simulink model "State_Feedback_NON_Linear_ROS"  (R2022b)
settings: Solver=FixedStepAuto  StartTime=0.0  StopTime=45  FixedStep=0.02  RelTol=1e-3
undefined symbols (not defined in the file): unicycle, X, Y
libraries: robotlib x3, simulink_extras x2
settings Model: Creator=Musta  LastModifiedBy=Musta
settings OptimizationCC: EnhancedBackFolding=on  PassReuseOutputArgsAs=Individual arguments  ZeroExternalMemoryAtStartup=off  ZeroInternalMemoryAtStartup=off  MaxStackSize=64  OptimizeBlockOrder=speed  DifferentSizesBufferReuse=on  OptimizationCustomize=off  EfficientTunableParamExpr=on
settings DebuggingCC: ParameterTunabilityLossMsg=error
settings HardwareCC: ProdBitPerPointer=32  ProdBitPerSizeT=32  ProdBitPerPtrDiffT=32  ProdLargestAtomicFloat=None  ProdIntDivRoundTo=Undefined  ProdEndianess=Unspecified  ProdWordSize=32  ProdHWDeviceType=Generic->Unspecified (assume 32-bit Generic)
settings SFSimCC: MATLABDynamicMemAlloc=off
settings RTWCC: Description=Embedded Coder  SystemTargetFile=ert.tlc  HardwareBoard=Robot Operating System (ROS)  TLCOptions="-aInlineSetEventsForThisBaseRateFcn=TLC_FALSE -aSuppressMultiTaskScheduler=TLC_FALSE  -aRateBasedStepFcn=0"  TemplateMakefile=ert_default_tmf  Toolchain=Catkin  TargetLang=C++
settings CodeAppCC: ForceParamTrailComments=on  IgnoreCustomStorageClasses=off  OperatorAnnotations=on  SimulinkDataObjDesc=on  SFDataObjDesc=on  InsertBlockDesc=on

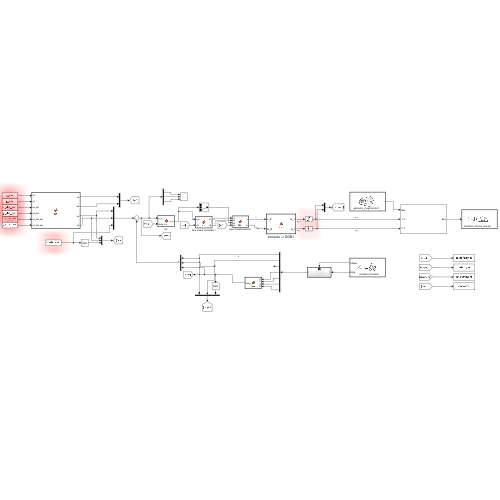
[thumbnail: Simulink's stored preview of the top-level diagram]
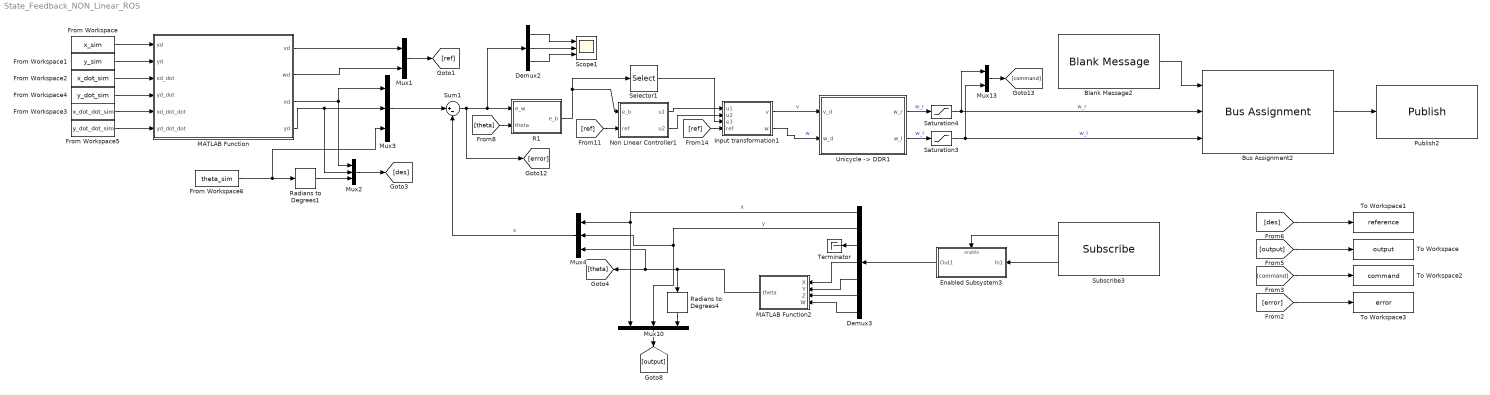
== system State_Feedback_NON_Linear_ROS ==
  Blank Message2 : robotlib/Blank Message  messageClass=Message  entityType=geometry_msgs/Vector3  messageType=geometry_msgs/Vector3  SampleTime=0.02  legacyBusStruct=off
      settings: LibrarySourceBlock=roslib/ROS/Blank Message
  Bus Assignment2 : BusAssignment  AssignedSignals=X,Y
  Demux2 : Demux  Outputs=3
  Demux3 : Demux  Outputs=7
  Enabled Subsystem3 : Subsystem  TreatAsAtomicUnit=on
  From Workspace : FromWorkspace  VariableName=x_sim
  From Workspace1 : FromWorkspace  VariableName=y_sim
  From Workspace2 : FromWorkspace  VariableName=x_dot_sim
  From Workspace3 : FromWorkspace  VariableName=x_dot_dot_sim
  From Workspace4 : FromWorkspace  VariableName=y_dot_sim
  From Workspace5 : FromWorkspace  VariableName=y_dot_dot_sim
  From Workspace6 : FromWorkspace  VariableName=theta_sim
  Input transformation1 : MATLAB Function  TreatAsAtomicUnit=on
  MATLAB Function : MATLAB Function  TreatAsAtomicUnit=on
  MATLAB Function2 : MATLAB Function  TreatAsAtomicUnit=on
  Mux1 : Mux  Inputs=2
  Mux{2..4,10} (4 alike) : Mux  Inputs=3
  Mux13 : Mux  Inputs=2
  Non Linear Controller1 : MATLAB Function  TreatAsAtomicUnit=on
  Publish2 : robotlib/Publish  topicSource=Select from ROS network  topic=/turtlebot_03/cmd_wheels  messageType=geometry_msgs/Vector3  legacyBusStruct=off  messageQueueLength=1
      settings: LibrarySourceBlock=roslib/ROS/Publish
  R1 : MATLAB Function  TreatAsAtomicUnit=on
  Radians to Degrees1 : simulink_extras/Transformations/Radians to Degrees
  Radians to Degrees4 : simulink_extras/Transformations/Radians to Degrees
  Saturation3 : Saturate  UpperLimit=unicycle.omegaWheelMax  LowerLimit=unicycle.omegaWheelMin
  Saturation4 : Saturate  UpperLimit=unicycle.omegaWheelMax  LowerLimit=unicycle.omegaWheelMin
  Scope1 : Scope  NumInputPorts=3
  Selector1 : Selector  InputPortWidth=3  IndexOptions=Index vector (dialog)  Indices=3  OutputSizes=1
  Subscribe3 : robotlib/Subscribe  topicSource=Select from ROS network  topic=/turtlebot_03/odom  messageType=nav_msgs/Odometry  SampleTime=0.02  legacyBusStruct=off  messageQueueLength=1
      settings: LibrarySourceBlock=roslib/ROS/Subscribe
  Sum1 : Sum  Inputs=|+-
  Terminator : Terminator
  To Workspace : ToWorkspace  VariableName=output  SaveFormat=Structure With Time  SampleTime=-1
  To Workspace1 : ToWorkspace  VariableName=reference  SaveFormat=Structure With Time  SampleTime=-1
  To Workspace2 : ToWorkspace  VariableName=command  SaveFormat=Structure With Time  SampleTime=-1
  To Workspace3 : ToWorkspace  VariableName=error  SaveFormat=Structure With Time  SampleTime=-1
  "Unicycle -> DDR1" : MATLAB Function  TreatAsAtomicUnit=on
  wires:
  [command] -> To Workspace2/1
  [des] -> To Workspace1/1
  [output] -> To Workspace/1
  [error] -> To Workspace3/1
  Subscribe3/2 -> Enabled Subsystem3/1(In1)
  Subscribe3/1 -> Enabled Subsystem3/Enable
  Demux2/2 -> Scope1/2
  Non Linear Controller1/1(u1) -> Input transformation1/1(u1)
  [theta] -> R1/2(theta)
  Demux2/1 -> Scope1/1
  Sum1/1 -> [error], R1/1(e_w), Demux2/1
  Blank Message2/1 -> Bus Assignment2/1
  Input transformation1/1(v) -> "Unicycle -> DDR1"/1(v_d)  "v"
  Selector1/1 -> Input transformation1/3(e3)
  [ref] -> Non Linear Controller1/2(ref)
  Input transformation1/2(w) -> "Unicycle -> DDR1"/2(w_d)  "w"
  Mux13/1 -> [command]
  Saturation4/1 -> Bus Assignment2/2, Mux13/1  "w_r"
  Demux2/3 -> Scope1/3
  Saturation3/1 -> Bus Assignment2/3, Mux13/2  "w_l"
  R1/1(e_b) -> Non Linear Controller1/1(e_b), Selector1/1
  "Unicycle -> DDR1"/2(w_l) -> Saturation3/1  "w_l"
  [ref] -> Input transformation1/4(ref)
  Bus Assignment2/1 -> Publish2/1
  "Unicycle -> DDR1"/1(w_r) -> Saturation4/1  "w_r"
  Non Linear Controller1/2(u2) -> Input transformation1/2(u2)
  From Workspace/1 -> MATLAB Function/1("xd ")
  From Workspace6/1 -> Radians to Degrees1/1, Mux3/3
  Mux2/1 -> [des]
  Mux1/1 -> [ref]
  MATLAB Function/2(wd) -> Mux1/2
  From Workspace1/1 -> MATLAB Function/2("yd ")
  From Workspace3/1 -> MATLAB Function/5(xd_dot_dot)
  From Workspace5/1 -> MATLAB Function/6(yd_dot_dot)
  MATLAB Function/4(yd) -> Mux2/2, Mux3/2
  From Workspace2/1 -> MATLAB Function/3(xd_dot)
  From Workspace4/1 -> MATLAB Function/4(yd_dot)
  MATLAB Function/1(vd) -> Mux1/1
  Mux3/1 -> Sum1/1
  Radians to Degrees1/1 -> Mux2/3
  MATLAB Function/3(xd) -> Mux3/1, Mux2/1
  MATLAB Function2/1(theta) -> Radians to Degrees4/1, Mux4/3, [theta]
  Demux3/6 -> MATLAB Function2/3(Z)
  Enabled Subsystem3/1(Out1) -> Demux3/1
  Demux3/4 -> MATLAB Function2/1(X)
  Demux3/7 -> MATLAB Function2/4(W)
  Demux3/3 -> Terminator/1
  Demux3/5 -> MATLAB Function2/2(Y)
  Demux3/1 -> Mux4/1, Mux10/1  "x"
  Demux3/2 -> Mux4/2, Mux10/2  "y"
  Mux4/1 -> Sum1/2  "x"
  Mux10/1 -> [output]
  Radians to Degrees4/1 -> Mux10/3

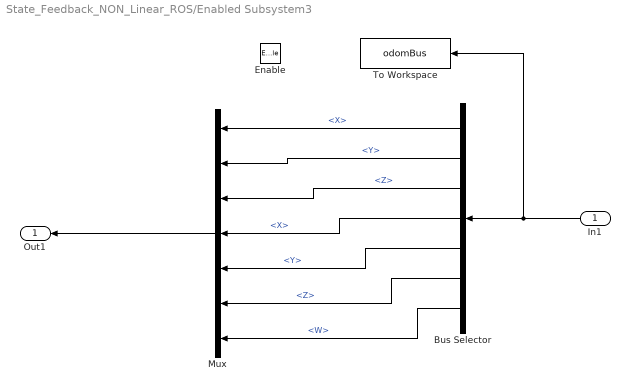
== system State_Feedback_NON_Linear_ROS/Enabled Subsystem3 ==
  In1 : Inport
  Enable : EnablePort
  Bus Selector : BusSelector  OutputSignals=Pose.Pose.Position.X,Pose.Pose.Position.Y,Pose.Pose.Position.Z,Pose.Pose.Orientation.X,Pose.Pose.Orientation.Y,Pose.Pose.Orientation.Z,Pose.Pose.Orientation.W
  Mux : Mux  Inputs=7
  To Workspace : ToWorkspace  VariableName=odomBus  SaveFormat=Timeseries  SampleTime=-1
  Out1 : Outport
  wires:
  Mux/1 -> Out1/1
  Bus Selector/1 -> Mux/1  "<X>"
  Bus Selector/2 -> Mux/2  "<Y>"
  In1/1 -> To Workspace/1, Bus Selector/1
  Bus Selector/3 -> Mux/3  "<Z>"
  Bus Selector/4 -> Mux/4  "<X>"
  Bus Selector/5 -> Mux/5  "<Y>"
  Bus Selector/6 -> Mux/6  "<Z>"
  Bus Selector/7 -> Mux/7  "<W>"

== matlab function State_Feedback_NON_Linear_ROS/Input transformation1 ==
  data: u1 input; v output; u2 input; e3 input; w output; ref input
function [v, w] = fcn(u1, u2, e3, ref)

    v = ref(1)*cos(e3) - u1;
    w = ref(2) - u2;

end

== matlab function State_Feedback_NON_Linear_ROS/MATLAB Function ==
  data: xd input; vd output; yd input; xd_dot input; yd_dot input; xd_dot_dot input; yd_dot_dot input; wd output; xd output; yd output
function [vd, wd, xd, yd] = fcn(xd, yd, xd_dot, yd_dot, xd_dot_dot, yd_dot_dot)
    
    vd = sqrt(xd_dot.^2 + yd_dot.^2);
    wd = (xd_dot.*yd_dot_dot - xd_dot_dot.*yd_dot) / (xd_dot.^2 + yd_dot.^2);

    xd = xd;
    yd = yd;

end

== matlab function State_Feedback_NON_Linear_ROS/Non Linear Controller1 ==
  data: e_b input; u1 output; ref input; u2 output
function [u1,u2] = fcn(e_b, ref)

    %#codegen
    coder.extrinsic('evalin')
    a = 0;                  % Needed in order to set variable class correctly
    zeta = 0;                  % Needed in order to set variable class correctly
    a = evalin('base','a'); % Read value from workspace
    zeta = evalin('base','zeta'); % Read value from workspace

    b = (a^2 - ref(2)^2) / ref(1);

    k1 = 2*zeta*sqrt(b*ref(1) + ref(2)^2);
    k2 = b;
    k3 = 2*zeta*sqrt(b*ref(1) + ref(2)^2);

    u1 = -k1*e_b(1);
    u2 = (-k2*ref(1)*sin(e_b(3))*e_b(2)) / e_b(3)  -k3*e_b(3);

end

== matlab function State_Feedback_NON_Linear_ROS/R1 ==
  data: e_w input; e_b output; theta input
function e_b  = fcn(e_w, theta)
    
    R = [cos(theta), sin(theta), 0;
        -sin(theta), cos(theta), 0;
         0, 0, 1];

    e_b = R * e_w;

end

== matlab function State_Feedback_NON_Linear_ROS/Unicycle -> DDR1 ==
  data: v_d input; w_r output; w_d input; w_l output
function [w_r, w_l] = fcn(v_d, w_d)

    %#codegen
    coder.extrinsic('evalin')
    d = 0;                  % Needed in order to set variable class correctly
    r = 0;                  % Needed in order to set variable class correctly
    d = evalin('base','unicycle.d'); % Read value from workspace
    r = evalin('base','unicycle.r'); % Read value from workspace

    w_r = ((2 * v_d) + (w_d * d)) / (2 * r);
    w_l = ((2 * v_d) - (w_d * d)) / (2 * r);

end

== matlab function State_Feedback_NON_Linear_ROS/MATLAB Function2 ==
  data: X input; theta output; Y input; Z input; W input
function theta = fcn(X, Y, Z, W)

    q_x = X;
    q_y = Y;
    q_z = Z;
    q_w = W;
    
    q = cat(2,q_x,q_y,q_z,q_w); 
    eulZYX = quat2eul(q,'ZYX');
    theta = eulZYX(:,3);
    
end
